simulink model "HW10_111205023"  (R2022b)
settings: Solver=VariableStepAuto  StartTime=0.0  StopTime=inf  RelTol=1e-3
libraries: commsync2 x2, commdigbbndpm3 x2, commfilt2 x2, commchan3 x1, commrandsrc3 x1, simulink x1, commrflib2 x1, dspsigops x1
settings Model: Creator=User  LastModifiedBy=User

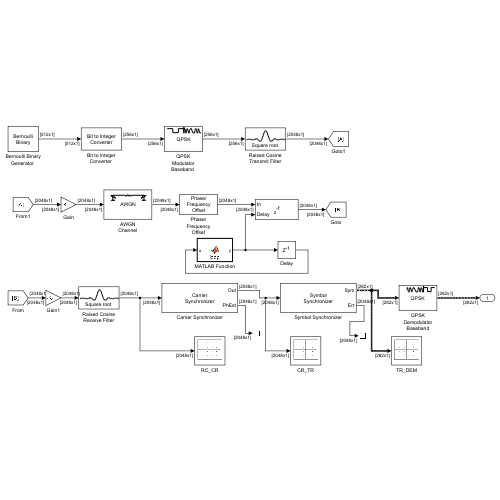
[thumbnail: Simulink's stored preview of the top-level diagram]
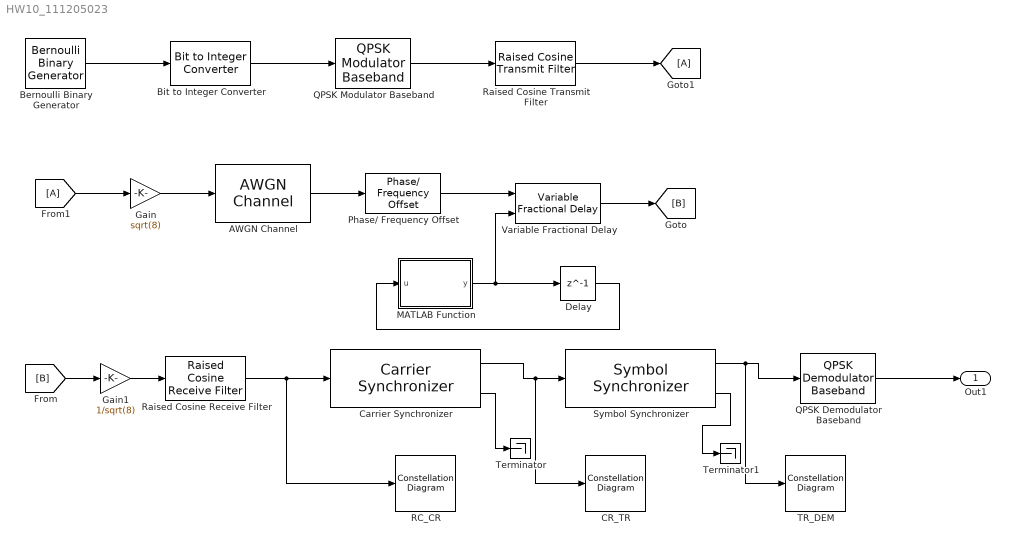
== system HW10_111205023 ==
  AWGN Channel : commchan3/AWGN Channel  InputProcessing=Columns as channels (frame based)  seed=61  noiseMode="Signal to noise ratio  (Eb/No)"  EbNodB=20  EsNodB=10  SNRdB=10  bitsPerSym=1  Ps=1  Tsym=1  variance=1
  "Bernoulli Binary Generator " : commrandsrc3/Bernoulli Binary Generator  ProbabilityOfZero=0.5  SeedSource=Parameter  Seed=61  SampleTime=1  SamplesPerFrame=512  OutputDataType=double  SimulateUsing=Interpreted execution
  "Bit to Integer Converter " : simulink/Logic and Bit Operations/Bit to Integer Converter  nbits=2  bitOrder=MSB first  signedOutputValues=Unsigned  outDtype=Inherit via internal rule  outDtypeSigned=Inherit via internal rule
  CR_TR : ConstellationDiagram  WindowPosition=[586.000000,119.000000,600.000000,596.000000,]  Visible=on  ScopeFrameLocation=window  XLimits=[-1.47,1.47]  YLimits=[-1.38,1.38]
  Carrier Synchronizer : commsync2/Carrier Synchronizer  Modulation=QPSK  ModulationPhaseOffset=Auto  CustomPhaseOffset=0  SamplesPerSymbol=8  DampingFactor=0.707  NormalizedLoopBandwidth=0.01  EstimatedPhaseErrorOutputPort=on  SimulateUsing=Interpreted execution
  Delay : Delay  DelayLength=1  InitialCondition=0
  From1 : From
  Gain : Gain  Gain=sqrt(8)
  Gain1 : Gain  Gain=1/sqrt(8)
  Goto1 : Goto
  MATLAB Function : MATLAB Function  TreatAsAtomicUnit=on
  Phase/ Frequency Offset : commrflib2/Phase// Frequency Offset  phaseOffset=0  freqPort=off  freqOffset=4e-3
  QPSK Demodulator Baseband : commdigbbndpm3/QPSK Demodulator Baseband  OutType=Integer  DecType=Hard decision  VarSource=Dialog  Variance=1  Dec=Gray  Ph=pi/4  outDtype1=Inherit via internal rule  outDtype2=Inherit via internal rule  derotateFactorWordLen=16  derotateFactorDataTypeStr=Inherit: Same word length as input  derotateFactorLastDataTypeStr=Inherit: Same word length as input
  "QPSK Modulator Baseband " : commdigbbndpm3/QPSK Modulator Baseband  InType=Integer  Enc=Gray  Ph=pi/4  outDtype=double  outWordLen=16  outUDDataType=sfix(16)  outFracLenMode=Best precision  outFracLen=15  outDataTypeStr=double  outLastDataTypeStr=double
  RC_CR : ConstellationDiagram  WindowPosition=[54.000000,118.000000,600.000000,600.000000,]  Visible=on  ScopeFrameLocation=window  XLimits=[-1.46,1.46]  YLimits=[-1.38,1.38]
  Raised Cosine Receive Filter : commfilt2/Raised Cosine Receive Filter  filtType=Square root  R=0.3  filtSpan=10  N=8  downFactor=1  downOffset=0  filterGain=1  InputProcessing=Columns as channels (frame based)  RateOptions=Allow multirate processing  framing=Mute  checkCoeff=off  variableName=rcRxFilt  currentFiltSpan=10  D=5  inputOffset=0  sampMode=Mute  saveAsFlag=0  rateMode=Downsampling  checkGain=Normalized  launchFVT=on  roundingMode=Floor  overflowMode=off  coeffDataTypeStr=Inherit: Same word length as input  coeffMin=[]  coeffMax=[]  coeffLastDataTypeStr=Inherit: Same word length as input  accumDataTypeStr=Inherit: Same as product output  accumLastDataTypeStr=Inherit: Same as product output  outputDataTypeStr=Inherit: Same as accumulator  outputMin=[]  outputMax=[]  outputLastDataTypeStr=Inherit: Same as accumulator
      settings: LibrarySourceBlock=|
      | commhdlfilt/Raised Cosine
      | Receive Filter
  Raised Cosine Transmit Filter : commfilt2/Raised Cosine Transmit Filter  filtType=Square root  R=0.3  filtSpan=10  N=8  filterGain=1  InputProcessing=Columns as channels (frame based)  RateOptions=Enforce single-rate processing  framing=Mute  checkCoeff=off  variableName=rcTxFilt  checkGain=Normalized  sampMode=Mute  saveAsFlag=0  currentFiltSpan=10  D=5  launchFVT=on  roundingMode=Floor  overflowMode=off  coeffDataTypeStr=Inherit: Same word length as input  coeffMin=[]  coeffMax=[]  coeffLastDataTypeStr=Inherit: Same word length as input  outputDataTypeStr=Inherit: Same as accumulator  outputMin=[]  outputMax=[]  outputLastDataTypeStr=Inherit: Same as accumulator
      settings: LibrarySourceBlock=|
      | commhdlfilt/Raised Cosine
      | Transmit Filter
  Symbol Synchronizer : commsync2/Symbol Synchronizer  Modulation=PAM/PSK/QAM  TimingErrorDetector=Zero-Crossing (decision-directed)  SamplesPerSymbol=8  DampingFactor=1  NormalizedLoopBandwidth=0.01  DetectorGain=2.7  TimingErrorOutputPort=on  SimulateUsing=Interpreted execution
  TR_DEM : ConstellationDiagram  WindowPosition=[1139.000000,112.000000,600.000000,600.000000,]  Visible=on  ScopeFrameLocation=window
  Terminator : Terminator
  Terminator1 : Terminator
  Variable Fractional Delay : dspsigops/Variable Fractional Delay  mode=OBSOLETE  modeActive=Linear  L=4  FarrowL=4  R=10  alpha=1  dmax=100  InputProcessing=Columns as channels (frame based)  ic=0  noDFT=off  fallbackFIR=Clip to the minimum value necessary for centered kernel  fallbackFarrow=Clip to the minimum value necessary for centered kernel  roundingMode=Zero  overflowMode=off
  Out1 : Outport
  wires:
  "Bernoulli Binary Generator "/1 -> "Bit to Integer Converter "/1
  "Bit to Integer Converter "/1 -> "QPSK Modulator Baseband "/1
  "QPSK Modulator Baseband "/1 -> Raised Cosine Transmit Filter/1
  Gain/1 -> AWGN Channel/1
  Phase/ Frequency Offset/1 -> Variable Fractional Delay/1
  MATLAB Function/1(y) -> Variable Fractional Delay/2, Delay/1
  Delay/1 -> MATLAB Function/1(u)
  AWGN Channel/1 -> Phase/ Frequency Offset/1
  Variable Fractional Delay/1 -> [B]
  Raised Cosine Receive Filter/1 -> RC_CR/1, Carrier Synchronizer/1
  Carrier Synchronizer/1 -> CR_TR/1, Symbol Synchronizer/1
  Raised Cosine Transmit Filter/1 -> Goto1/1
  From1/1 -> Gain/1
  Symbol Synchronizer/1 -> TR_DEM/1, QPSK Demodulator Baseband/1
  QPSK Demodulator Baseband/1 -> Out1/1
  Gain1/1 -> Raised Cosine Receive Filter/1
  [B] -> Gain1/1
  Carrier Synchronizer/2 -> Terminator/1
  Symbol Synchronizer/2 -> Terminator1/1

== matlab function HW10_111205023/MATLAB Function ==
  data: u input; y output
function y = loop(u)
    y = u+0.001;
end
